simulink model "diagramas"  (R2014a)
settings: Solver=ode45  StartTime=0.0  StopTime=10.0  RelTol=1e-6
libraries: fl_lib x39, nesl_utility x3
settings Model: Creator=kikez  LastModifiedBy=jose6alejandro

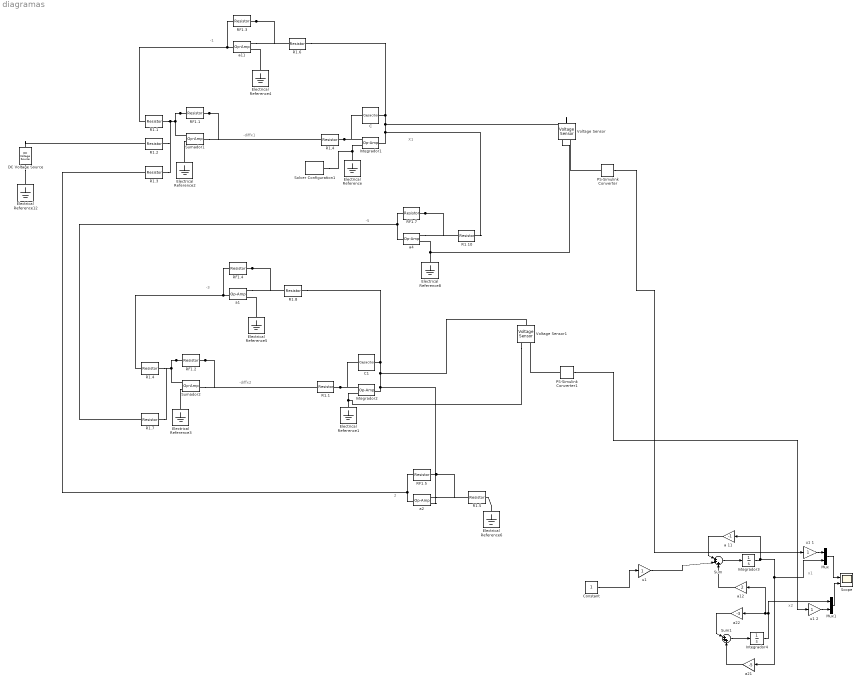
== system diagramas ==
  note: 2
  note: -5
  note: -1
  note: -diffx1
  note: X1
  note: -3
  note: -diffx2
  note: x2
  note: x1
  C : fl_lib/Electrical/Electrical Elements/Capacitor  c=0.1e-6 F  r=0 Ohm  g=0 1/Ohm  i_specify=off  i_priority=High  i=0 A  v_specify=off  v_priority=High  v=0 V  vc_specify=off  vc_priority=High  vc=0 V
  C1 : fl_lib/Electrical/Electrical Elements/Capacitor  c=0.1e-6 F  r=0 Ohm  g=0 1/Ohm  i_specify=off  i_priority=High  i=0 A  v_specify=off  v_priority=High  v=0 V  vc_specify=off  vc_priority=High  vc=0 V
  Constant : Constant
  DC Voltage Source : fl_lib/Electrical/Electrical Sources/DC Voltage Source  v0=1 V
  Electrical Reference{,1..6,8,12} (9 alike) : fl_lib/Electrical/Electrical Elements/Electrical Reference
  Integrador1 : fl_lib/Electrical/Electrical Elements/Op-Amp  outI_specify=off  outI_priority=High  outI=0 A
  Integrador2 : fl_lib/Electrical/Electrical Elements/Op-Amp  outI_specify=off  outI_priority=High  outI=0 A
  Integrador3 : Integrator
  Integrador4 : Integrator
  Mux : Mux  Inputs=2
  Mux1 : Mux  Inputs=2
  PS-Simulink Converter : nesl_utility/PS-Simulink Converter  PhysicalDomain=network_engine_domain  SubClassName=ps_output  LeftPortType=input  RightPortType=output  PseudoPeriodic=off  Frequencies=[]  Unit=1  AffineConversion=off
  PS-Simulink Converter1 : nesl_utility/PS-Simulink Converter  PhysicalDomain=network_engine_domain  SubClassName=ps_output  LeftPortType=input  RightPortType=output  PseudoPeriodic=off  Frequencies=[]  Unit=1  AffineConversion=off
  R1,1 : fl_lib/Electrical/Electrical Elements/Resistor  R=10 MOhm  i_specify=off  i_priority=High  i=0 A  v_specify=off  v_priority=High  v=0 V
  R1,4 : fl_lib/Electrical/Electrical Elements/Resistor  R=10 MOhm  i_specify=off  i_priority=High  i=0 A  v_specify=off  v_priority=High  v=0 V
  R1.{1..8,10} (9 alike) : fl_lib/Electrical/Electrical Elements/Resistor  R=1000 Ohm  i_specify=off  i_priority=High  i=0 A  v_specify=off  v_priority=High  v=0 V
  RF1.{1..3,5} (4 alike) : fl_lib/Electrical/Electrical Elements/Resistor  R=1000 Ohm  i_specify=off  i_priority=High  i=0 A  v_specify=off  v_priority=High  v=0 V
  RF1.4 : fl_lib/Electrical/Electrical Elements/Resistor  R=3000 Ohm  i_specify=off  i_priority=High  i=0 A  v_specify=off  v_priority=High  v=0 V
  RF1.7 : fl_lib/Electrical/Electrical Elements/Resistor  R=5000 Ohm  i_specify=off  i_priority=High  i=0 A  v_specify=off  v_priority=High  v=0 V
  Scope : Scope  NumInputPorts=2
      settings: TimeRange=10  YMin=0~-0.45  YMax=0.35~0
  Solver Configuration1 : nesl_utility/Solver Configuration  PhysicalDomain=network_engine_domain  SubClassName=solver  LeftPortType=input  RightPortType=generic  Accelerate=off  Tones=[]  Harmonics=[]  SimulateNoise=off  Profile=off  UseLocalSampling=off  EnableSwitchedLinearOptims=on  FrequencyDomain=off  UseCCode=off  RelTol=0.001  AbsTol=1e-06  MinStep=1e-09  ToWorkspace=off  DoDC=off  ResidualTolerance=1e-09  UseLocalSolver=off  LocalSolverChoice=NE_BACKWARD_EULER_ADVANCER  LocalSolverSampleTime=0.001  DoFixedCost=off  MaxNonlinIter=3  MaxModeIter=2  LinearAlgebra=Sparse  DelaysMemoryBudget=1024  AutomaticFiltering=on  FilteringTimeConstant=0.001
  Sum : Sum  Inputs=|+++
  Sum1 : Sum  Inputs=|+++
  "Sumador1 " : fl_lib/Electrical/Electrical Elements/Op-Amp  outI_specify=off  outI_priority=High  outI=0 A
  Sumador2 : fl_lib/Electrical/Electrical Elements/Op-Amp  outI_specify=off  outI_priority=High  outI=0 A
  Voltage Sensor : fl_lib/Electrical/Electrical Sensors/Voltage Sensor
  Voltage Sensor1 : fl_lib/Electrical/Electrical Sensors/Voltage Sensor
  a 11 : Gain  Gain=-1
  a{1..2,4,11} (4 alike) : fl_lib/Electrical/Electrical Elements/Op-Amp  outI_specify=off  outI_priority=High  outI=0 A
  a12 : Gain  Gain=2
  a21 : Gain  Gain=-5
  "a22 " : Gain  Gain=-3
  "u1 " : Gain
  u1 1 : Gain
  u1 2 : Gain
  wires:
  Constant/1 -> "u1 "/1
  Sum/1 -> Integrador3/1
  a 11/1 -> Sum/1
  "u1 "/1 -> Sum/2
  Sum1/1 -> Integrador4/1
  "a22 "/1 -> Sum1/1
  Integrador3/1 -> Mux/2, a21/1, a 11/1
  a21/1 -> Sum1/3
  a12/1 -> Sum/3
  Integrador4/1 -> Mux1/1, a12/1, "a22 "/1
  PS-Simulink Converter1/1 -> u1 2/1
  PS-Simulink Converter/1 -> u1 1/1
  u1 1/1 -> Mux/1
  u1 2/1 -> Mux1/2
  Mux1/1 -> Scope/2
  Mux/1 -> Scope/1
  connections:
  RF1.1/LConn1 -- "Sumador1 "/LConn2 -- R1.2/RConn1 -- R1.3/RConn1 -- R1.1/RConn1
  RF1.1/RConn1 -- R1,4/LConn1 -- "Sumador1 "/RConn1
  Electrical Reference2/LConn1 -- "Sumador1 "/LConn1
  R1,4/RConn1 -- Integrador1/LConn2 -- C/LConn1
  Electrical Reference/LConn1 -- Solver Configuration1/RConn1 -- Integrador1/LConn1
  DC Voltage Source/RConn1 -- Electrical Reference12/LConn1
  DC Voltage Source/LConn1 -- R1.2/LConn1
  RF1.3/LConn1 -- a11/LConn2 -- R1.6/LConn1
  RF1.3/RConn1 -- R1.1/LConn1 -- a11/RConn1
  Electrical Reference4/LConn1 -- a11/LConn1
  R1.6/RConn1 -- Voltage Sensor/LConn1 -- R1.10/RConn1 -- Integrador1/RConn1 -- C/RConn1
  RF1.2/LConn1 -- Sumador2/LConn2 -- R1.7/RConn1 -- R1.4/RConn1
  RF1.2/RConn1 -- R1,1/LConn1 -- Sumador2/RConn1
  R1,1/RConn1 -- Integrador2/LConn2 -- C1/LConn1
  RF1.4/LConn1 -- a1/LConn2 -- R1.8/LConn1
  a1/RConn1 -- RF1.4/RConn1 -- R1.4/LConn1
  R1.8/RConn1 -- Voltage Sensor1/LConn1 -- a2/LConn1 -- Integrador2/RConn1 -- C1/RConn1
  Electrical Reference5/LConn1 -- a1/LConn1
  Electrical Reference1/LConn1 -- Voltage Sensor1/RConn2 -- Integrador2/LConn1
  Electrical Reference3/LConn1 -- Sumador2/LConn1
  RF1.5/LConn1 -- a2/LConn2 -- R1.5/LConn1
  RF1.5/RConn1 -- R1.3/LConn1 -- a2/RConn1
  RF1.7/LConn1 -- a4/LConn2 -- R1.10/LConn1
  RF1.7/RConn1 -- R1.7/LConn1 -- a4/RConn1
  Electrical Reference8/LConn1 -- Voltage Sensor/RConn2 -- a4/LConn1
  PS-Simulink Converter/LConn1 -- Voltage Sensor/RConn1
  PS-Simulink Converter1/LConn1 -- Voltage Sensor1/RConn1
  Electrical Reference6/LConn1 -- R1.5/RConn1
